simulink model "PID_Controller"  (R2014b)
settings: Solver=ode4  StartTime=0.0  StopTime=30  FixedStep=0.001  RelTol=1e-3
undefined symbols (not defined in the file): Advantech, PCI
libraries: rtwinlib x2, fuzblock x1
settings Model: SimulationMode=external  ExtModeTrigDuration=200000  Creator=Administrator  LastModifiedBy=nk
settings DataIOCC: SignalLoggingSaveFormat=ModelDataLogs
settings OptimizationCC: ExpressionDepthLimit=2147483647  InitFltsAndDblsToZero=on
settings DebuggingCC: SaveWithParameterizedLinksMsg=none  UnderspecifiedInitializationDetection=Classic  MergeDetectMultiDrivingBlocksExec=none  SignalResolutionControl=TryResolveAllWithWarning  MultiTaskDSMMsg=warning  MultiTaskCondExecSysMsg=none  FcnCallInpInsideContextMsg=UseLocalSettings  StateNameClashWarn=warning
settings RTWCC: SystemTargetFile=rtwin.tlc  TemplateMakefile=rtwin.tmf  Description=Real-Time Windows Target  ProcessScript=rtwin_make_rtw_hook  IncludeERTFirstTime=on
settings RTWinTargetCC: TargetFcnLib=ansi_tfl_tmw.mat  TargetLibSuffix=_rtwin.lib  TargetPreCompLibLocation=C:\Program Files\MATLAB\R2014b\toolbox\rtw\targets\rtwin\lib\win64  ModelReferenceCompliant=off  CompOptLevelCompliant=off

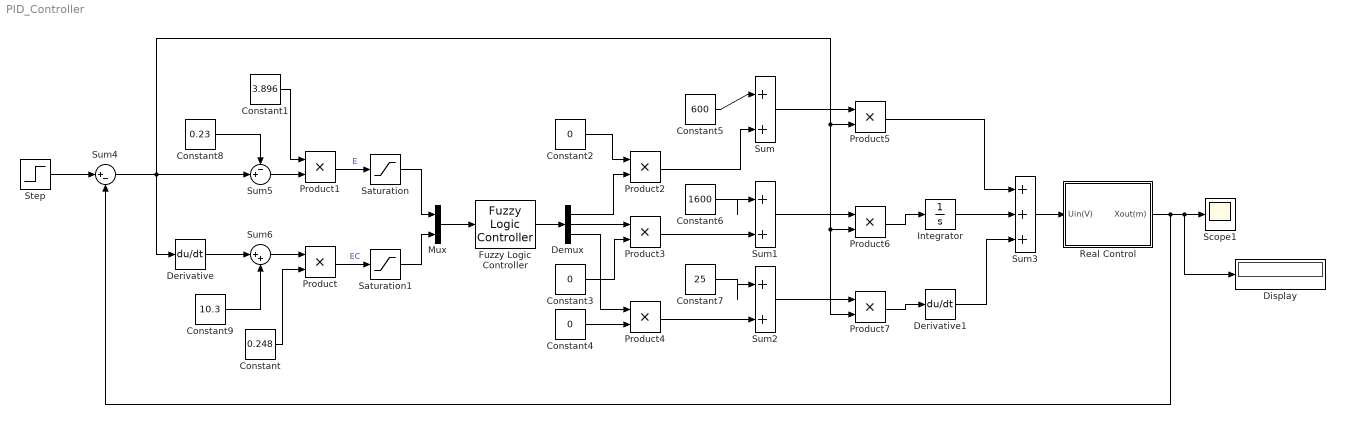
== system PID_Controller ==
  Constant : Constant  Value=0.248
  Constant1 : Constant  Value=3.896
  Constant2 : Constant  Value=0
  Constant3 : Constant  Value=0
  Constant4 : Constant  Value=0
  Constant5 : Constant  Value=600
  Constant6 : Constant  Value=1600
  Constant7 : Constant  Value=25
  Constant8 : Constant  Value=0.23
  Constant9 : Constant  Value=10.3
  Demux : Demux  Outputs=3
  Derivative : Derivative
  Derivative1 : Derivative
  Display : Display
  Fuzzy Logic Controller : fuzblock/Fuzzy Logic  Controller  fis=fzy
  Integrator : Integrator
  Mux : Mux  Inputs=2
  Product{,1..7} (8 alike) : Product
  Real Control : Subsystem
  Saturation : Saturate
  Saturation1 : Saturate
  Scope1 : Scope
      settings: YMin=-0.013  YMax=-0.009  SaveName=None  MaxDataPoints=500000000
  Step : Step  Time=15  Before=-0.01  After=-0.011  SampleTime=0
  Sum{,1..2,6} (4 alike) : Sum  Inputs=|++
  Sum3 : Sum  Inputs=+++
  Sum4 : Sum  Inputs=|+-
  Sum5 : Sum  Inputs=-+|
  wires:
  Constant1/1 -> Product1/1
  Sum4/1 -> Sum5/2, Derivative/1, Product7/2, Product6/2, Product5/2
  Constant/1 -> Product/2
  Product1/1 -> Saturation/1  "E"
  Product/1 -> Saturation1/1  "EC"
  Saturation/1 -> Mux/1
  Saturation1/1 -> Mux/2
  Mux/1 -> Fuzzy Logic Controller/1
  Fuzzy Logic Controller/1 -> Demux/1
  Demux/1 -> Product2/2
  Demux/2 -> Product3/1
  Demux/3 -> Product4/1
  Constant2/1 -> Product2/1
  Constant3/1 -> Product3/2
  Constant4/1 -> Product4/2
  Constant5/1 -> Sum/1
  Product2/1 -> Sum/2
  Constant6/1 -> Sum1/1
  Product3/1 -> Sum1/2
  Constant7/1 -> Sum2/1
  Product4/1 -> Sum2/2
  Sum/1 -> Product5/1
  Sum1/1 -> Product6/1
  Sum2/1 -> Product7/1
  Product5/1 -> Sum3/1
  Product6/1 -> Integrator/1
  Integrator/1 -> Sum3/2
  Product7/1 -> Derivative1/1
  Derivative1/1 -> Sum3/3
  Step/1 -> Sum4/1
  Sum3/1 -> Real Control/1(Uin(V))
  Real Control/1(Xout(m)) -> Sum4/2, Display/1, Scope1/1
  Sum5/1 -> Product1/2
  Constant8/1 -> Sum5/1
  Constant9/1 -> Sum6/2
  Derivative/1 -> Sum6/1
  Sum6/1 -> Product/1

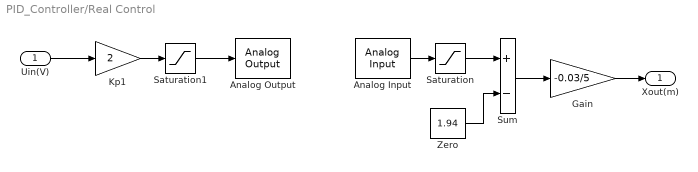
== system PID_Controller/Real Control ==
  Uin(V) : Inport
  Analog Input : rtwinlib/Analog Input  SampleTime=0.001  MaxMissedTicks=10  ShowMissedTicks=off  YieldWhenWaiting=off  DrvName=Advantech/PCI-1711  DrvAddress=4294967295  DrvOptions=zeros(1,0)  Channels=1  RangeMode=1  VoltRange=2  DataType=1
      settings: AttributesFormatString=Advantech\nPCI-1711 [auto]
  Analog Output : rtwinlib/Analog Output  SampleTime=0.001  MaxMissedTicks=10  ShowMissedTicks=off  YieldWhenWaiting=off  DrvName=Advantech/PCI-1711  DrvAddress=4294967295  DrvOptions=zeros(1,0)  Channels=1  RangeMode=1  VoltRange=2  InitialValue=-10  FinalValue=-10
      settings: AttributesFormatString=Advantech\nPCI-1711 [auto]
  Gain : Gain  Gain=-0.03/5  SaturateOnIntegerOverflow=on  OutDataTypeStr=Inherit: Same as input  ParamDataTypeStr=Inherit: Same as input
  Kp1 : Gain  Gain=2  SaturateOnIntegerOverflow=on  OutDataTypeStr=Inherit: Same as input  ParamDataTypeStr=Inherit: Same as input
  Saturation : Saturate  UpperLimit=5  LowerLimit=0
  Saturation1 : Saturate  UpperLimit=10  LowerLimit=0
  Sum : Sum  Inputs=+-  SaturateOnIntegerOverflow=on  OutDataTypeStr=Inherit: Same as first input
  Zero : Constant  Value=1.94  SampleTime=-1
  Xout(m) : Outport
  wires:
  Gain/1 -> Xout(m)/1
  Zero/1 -> Sum/2
  Sum/1 -> Gain/1
  Saturation/1 -> Sum/1
  Analog Input/1 -> Saturation/1
  Kp1/1 -> Saturation1/1
  Uin(V)/1 -> Kp1/1
  Saturation1/1 -> Analog Output/1
